simulink model "ModeloSIR"  (R2021b)
settings: Solver=VariableStepAuto  StartTime=0.0  StopTime=100  MaxStep=0.1001  MinStep=0.100  RelTol=1e-3
values from neighbouring files (symbols this model uses):
  beta = X(2)    [ErroQuadratico.m]
  I0 = 1    [ErroQuadratico.m]
  r = X(1)    [ErroQuadratico.m]
  R0 = 0    [ErroQuadratico.m]
  S0 = 499    [ErroQuadratico.m]
settings Model: Creator=19.00565-2  LastModifiedBy=20.00601-2
settings SolverCC: InitialStep=0.1001

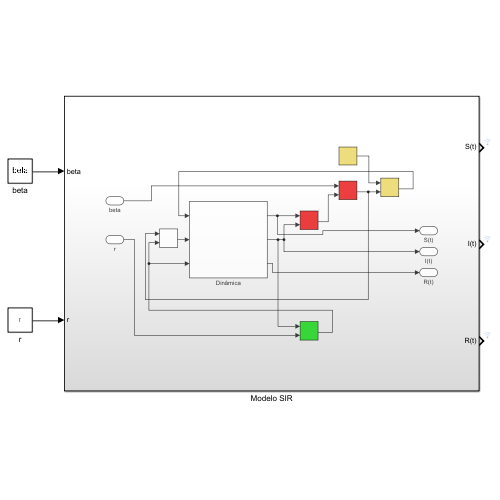
[thumbnail: Simulink's stored preview of the top-level diagram]
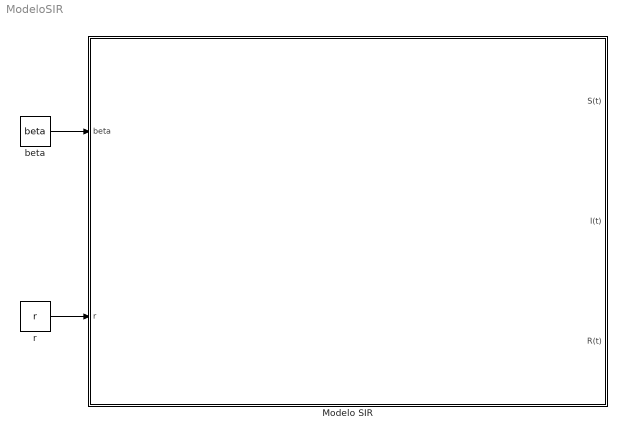
== system ModeloSIR ==
  Modelo SIR : Subsystem
  beta : Constant  Value=beta
  r : Constant  Value=r
  wires:
  r/1 -> Modelo SIR/2(r)
  beta/1 -> Modelo SIR/1(beta)

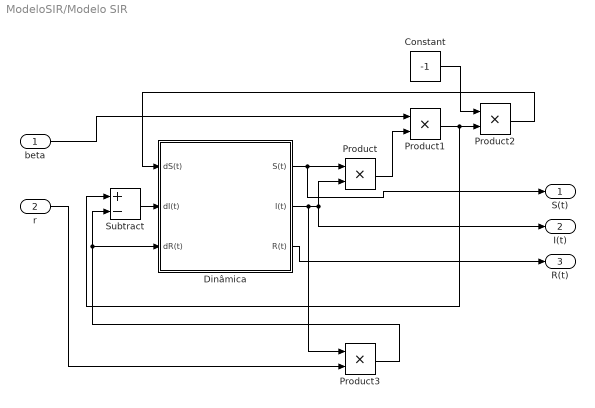
== system ModeloSIR/Modelo SIR ==
  beta : Inport
  r : Inport  Port=2
  Constant : Constant  Value=-1
  Dinâmica : Subsystem
  Product{,1..3} (4 alike) : Product
  Subtract : Sum  Inputs=+-
  S(t) : Outport
  I(t) : Outport  Port=2
  R(t) : Outport  Port=3
  wires:
  Constant/1 -> Product2/1
  Dinâmica/2(I(t)) -> Product3/1, I(t)/1, Product/2
  Product1/1 -> Subtract/1, Product2/2
  Product2/1 -> Dinâmica/1(dS(t))
  Dinâmica/1(S(t)) -> S(t)/1, Product/1
  r/1 -> Product3/2
  Product3/1 -> Dinâmica/3(dR(t)), Subtract/2
  Product/1 -> Product1/2
  Subtract/1 -> Dinâmica/2(dI(t))
  Dinâmica/3(R(t)) -> R(t)/1
  beta/1 -> Product1/1

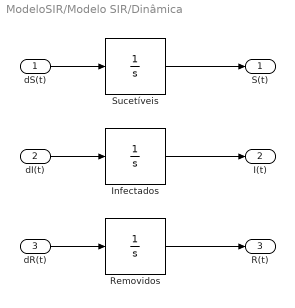
== system ModeloSIR/Modelo SIR/Dinâmica ==
  dS(t) : Inport
  dI(t) : Inport  Port=2
  dR(t) : Inport  Port=3
  Infectados : Integrator  InitialCondition=I0
  Removidos : Integrator  InitialCondition=R0
  Sucetíveis : Integrator  InitialCondition=S0
  S(t) : Outport
  I(t) : Outport  Port=2
  R(t) : Outport  Port=3
  wires:
  dR(t)/1 -> Removidos/1
  Sucetíveis/1 -> S(t)/1
  dI(t)/1 -> Infectados/1
  dS(t)/1 -> Sucetíveis/1
  Infectados/1 -> I(t)/1
  Removidos/1 -> R(t)/1
